simulink model "Doppelpendel_LQG"  (R2020b)
settings: Solver=ode45  StartTime=0.0  StopTime=10  EnableMultiTasking=on
values from neighbouring files (symbols this model uses):
  Beobachter_Rueckfuehrung = 0    [LoadParameter.m]
  Quantisierung = 0    [LoadParameter.m]
undefined symbols (not defined in the file or in its folder): parDP, parFF, parKAL, parLQR
libraries: cstblocks x3
settings Model: Creator=tg  LastModifiedBy=Armin Wessel
settings DataIOCC: LimitDataPoints=on  SaveFormat=Array  SignalLoggingSaveFormat=ModelDataLogs  ReturnWorkspaceOutputs=off
settings OptimizationCC: ExpressionDepthLimit=2147483647  InitFltsAndDblsToZero=on  LifeSpan=inf
settings DebuggingCC: UnderspecifiedInitializationDetection=Classic  MergeDetectMultiDrivingBlocksExec=none  SolverPrmCheckMsg=warning  FcnCallInpInsideContextMsg=warning  AllowSymbolicDim=off  StateNameClashWarn=warning  SFUnexpectedBacktrackingDiag=warning  SFNoUnconditionalDefaultTransitionDiag=warning  SFExecutionAtInitializationDiag=none  ArithmeticOperatorsInVariantConditions=warning
settings HardwareCC: ProdBitPerPointer=32  ProdBitPerSizeT=32  ProdBitPerPtrDiffT=32  ProdLargestAtomicFloat=None  ProdIntDivRoundTo=Undefined  ProdEndianess=Unspecified  ProdWordSize=32  ProdHWDeviceType=32-bit Generic
settings ModelReferenceCC: PropagateSignalLabelsOutOfModel=off
settings SFSimCC: SimUseLocalCustomCode=off  SimParseCustomCode=off  CustomCodeUndefinedFunction=UseInterfaceOnly
settings RTWCC: RTWUseLocalCustomCode=off
settings CodeAppCC: StateflowObjectComments=on
settings GRTTargetCC: TargetLangStandard=C89/C90 (ANSI)  CombineOutputUpdateFcns=off  GRTInterface=on
settings ConfigComp: CovMetricSettings=dw  CovSaveCumulativeToWorkspaceVar=on  CovSaveSingleToWorkspaceVar=on  CovExternalEMLEnable=off

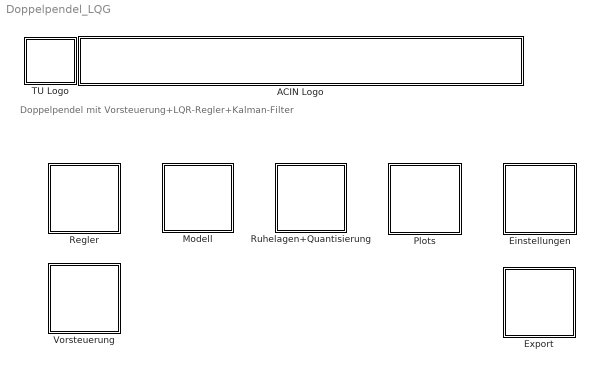
== system Doppelpendel_LQG ==
  note: Doppelpendel mit Vorsteuerung+LQR-Regler+Kalman-Filter
  ACIN Logo : Subsystem
      mask init:
      | s = get_param(gcb,'UserData');
      mask Display:
      | image(s.logo,[0 0 439 45]);
      | %axis image
  Einstellungen : Subsystem
  Export : Subsystem
  Modell : Subsystem
  Plots : Subsystem
  Regler : Subsystem
  Ruhelagen+Quantisierung : Subsystem
  TU Logo : Subsystem
      mask init:
      | s = get_param(gcb,'UserData');
      mask Display: image(s.logo,[0 0 45 45]);
  Vorsteuerung : Subsystem

== system Doppelpendel_LQG/ACIN Logo ==

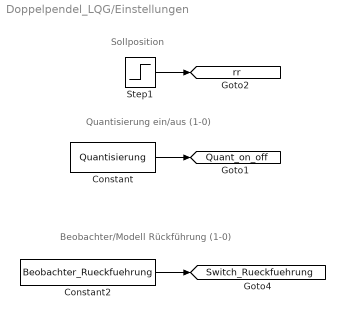
== system Doppelpendel_LQG/Einstellungen ==
  note: Sollposition
  note: Quantisierung ein/aus (1-0)
  note: Beobachter/Modell Rückführung (1-0)
  Constant : Constant  Value=Quantisierung
  Constant2 : Constant  Value=Beobachter_Rueckfuehrung
  Step1 : Step  After=0  SampleTime=parLQR.Ta
  tag scope: Quant_on_off=global, Switch_Rueckfuehrung=global, rr=global
  wires:
  Step1/1 -> [rr]
  Constant/1 -> [Quant_on_off]
  Constant2/1 -> [Switch_Rueckfuehrung]

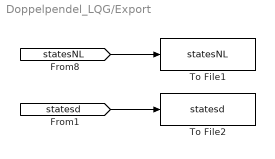
== system Doppelpendel_LQG/Export ==
  To File1 : ToFile  Filename=statesNL  MatrixName=data  SampleTime=parDP.Ta
  To File2 : ToFile  Filename=statesd  MatrixName=data  SampleTime=parDP.Ta
  wires:
  [statesNL] -> To File1/1
  [statesd] -> To File2/1

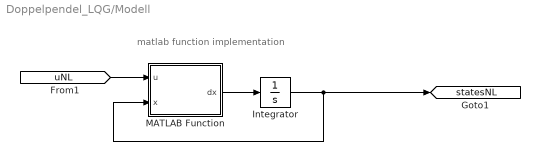
== system Doppelpendel_LQG/Modell ==
  note: matlab function implementation
  Integrator : Integrator  InitialCondition=parDP.IC
  MATLAB Function : MATLAB Function  TreatAsAtomicUnit=on
  tag scope: statesNL=global
  wires:
  [uNL] -> MATLAB Function/1(u)
  Integrator/1 -> [statesNL], MATLAB Function/2(x)
  MATLAB Function/1(dx) -> Integrator/1

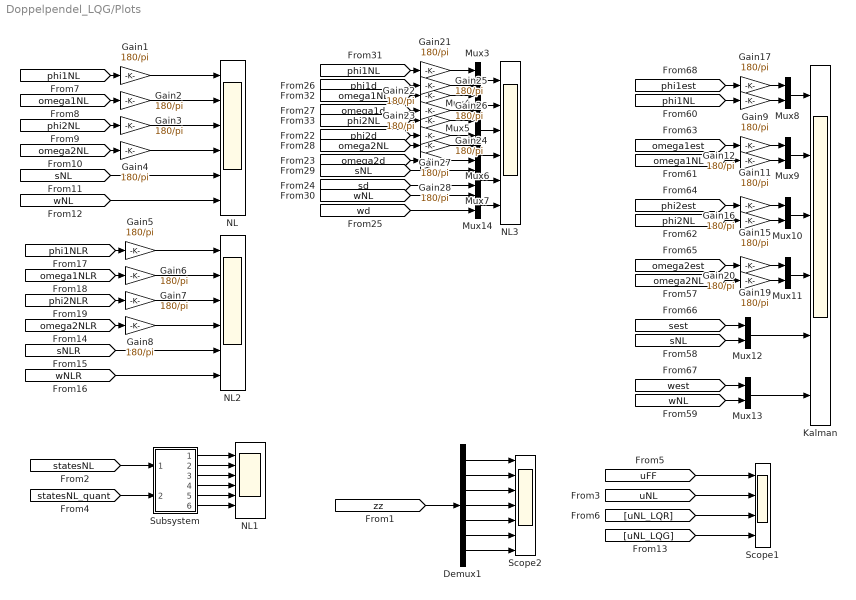
== system Doppelpendel_LQG/Plots ==
  Demux1 : Demux  Outputs=7
  Gain{1..9,11..12,15..17,19..28} (24 alike) : Gain  Gain=180/pi
  Kalman : Scope  NumInputPorts=6
  Mux{3..14} (12 alike) : Mux  Inputs=2
  NL{,1..3} (4 alike) : Scope  NumInputPorts=6
  Scope1 : Scope  NumInputPorts=4
  Scope2 : Scope  NumInputPorts=7
  Subsystem : Subsystem
  wires:
  [omega1NL] -> Gain2/1
  [omega2NL] -> Gain4/1
  [sNL] -> NL/5
  [wNL] -> NL/6
  Gain1/1 -> NL/1
  Gain2/1 -> NL/2
  Gain3/1 -> NL/3
  Gain4/1 -> NL/4
  [phi1NL] -> Gain1/1
  [phi2NL] -> Gain3/1
  [statesNL] -> Subsystem/1(In1)
  [statesNL_quant] -> Subsystem/2(In2)
  Subsystem/1(Out1) -> NL1/1
  Subsystem/2(Out2) -> NL1/2
  Subsystem/3(Out3) -> NL1/3
  Subsystem/4(Out4) -> NL1/4
  Subsystem/5(Out5) -> NL1/5
  Subsystem/6(Out6) -> NL1/6
  [omega1NL] -> Gain22/1
  [omega2NL] -> Gain24/1
  [phi1NL] -> Gain21/1
  [phi2NL] -> Gain23/1
  Mux3/1 -> NL3/1
  Mux4/1 -> NL3/2
  Mux5/1 -> NL3/3
  Mux6/1 -> NL3/4
  Mux7/1 -> NL3/5
  Mux14/1 -> NL3/6
  Gain21/1 -> Mux3/1
  Gain22/1 -> Mux4/1
  Gain23/1 -> Mux5/1
  Gain24/1 -> Mux6/1
  [sNL] -> Mux7/1
  [wNL] -> Mux14/1
  [phi1d] -> Gain25/1
  [omega1d] -> Gain26/1
  [phi2d] -> Gain27/1
  [omega2d] -> Gain28/1
  Gain25/1 -> Mux3/2
  Gain26/1 -> Mux4/2
  Gain27/1 -> Mux5/2
  Gain28/1 -> Mux6/2
  [sd] -> Mux7/2
  [wd] -> Mux14/2
  Demux1/1 -> Scope2/1
  Demux1/2 -> Scope2/2
  Demux1/3 -> Scope2/3
  Demux1/4 -> Scope2/4
  Demux1/5 -> Scope2/5
  Demux1/6 -> Scope2/6
  Demux1/7 -> Scope2/7
  [zz] -> Demux1/1
  Mux13/1 -> Kalman/6
  Mux12/1 -> Kalman/5
  Mux11/1 -> Kalman/4
  [omega1NL] -> Gain12/1
  [omega2NL] -> Gain20/1
  [phi1NL] -> Gain9/1
  [phi2NL] -> Gain16/1
  [sest] -> Mux12/1
  [west] -> Mux13/1
  [sNL] -> Mux12/2
  [wNL] -> Mux13/2
  Gain9/1 -> Mux8/2
  Gain17/1 -> Mux8/1
  [phi1est] -> Gain17/1
  Mux8/1 -> Kalman/1
  Gain12/1 -> Mux9/2
  Gain11/1 -> Mux9/1
  Mux9/1 -> Kalman/2
  [omega1est] -> Gain11/1
  Gain16/1 -> Mux10/2
  Gain15/1 -> Mux10/1
  [phi2est] -> Gain15/1
  Mux10/1 -> Kalman/3
  Gain20/1 -> Mux11/2
  Gain19/1 -> Mux11/1
  [omega2est] -> Gain19/1
  [uFF] -> Scope1/1
  [uNL] -> Scope1/2
  [uNL_LQR] -> Scope1/3
  [uNL_LQG] -> Scope1/4
  [omega1NLR] -> Gain6/1
  [omega2NLR] -> Gain8/1
  [sNLR] -> NL2/5
  [wNLR] -> NL2/6
  Gain5/1 -> NL2/1
  Gain6/1 -> NL2/2
  Gain7/1 -> NL2/3
  Gain8/1 -> NL2/4
  [phi1NLR] -> Gain5/1
  [phi2NLR] -> Gain7/1

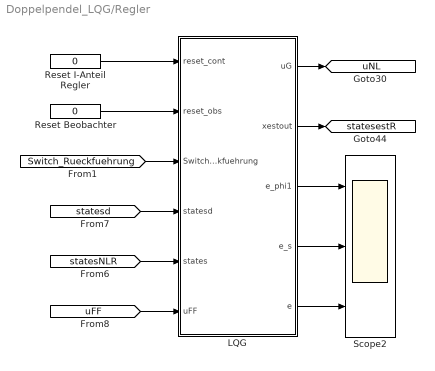
== system Doppelpendel_LQG/Regler ==
  LQG : MATLAB Function  TreatAsAtomicUnit=on
  Reset Beobachter : Constant  Value=0
  Reset I-Anteil Regler : Constant  Value=0
  Scope2 : Scope  NumInputPorts=3
  tag scope: statesestR=global, uNL=global
  wires:
  LQG/3(e_phi1) -> Scope2/1
  LQG/4(e_s) -> Scope2/2
  LQG/5(e) -> Scope2/3
  [statesNLR] -> LQG/5(states)
  LQG/2(xestout) -> [statesestR]
  [statesd] -> LQG/4(statesd)
  [uFF] -> LQG/6(uFF)
  LQG/1(uG) -> [uNL]
  Reset Beobachter/1 -> LQG/2(reset_obs)
  Reset I-Anteil Regler/1 -> LQG/1(reset_cont)
  [Switch_Rueckfuehrung] -> LQG/3(Switch_Rueckfuehrung)

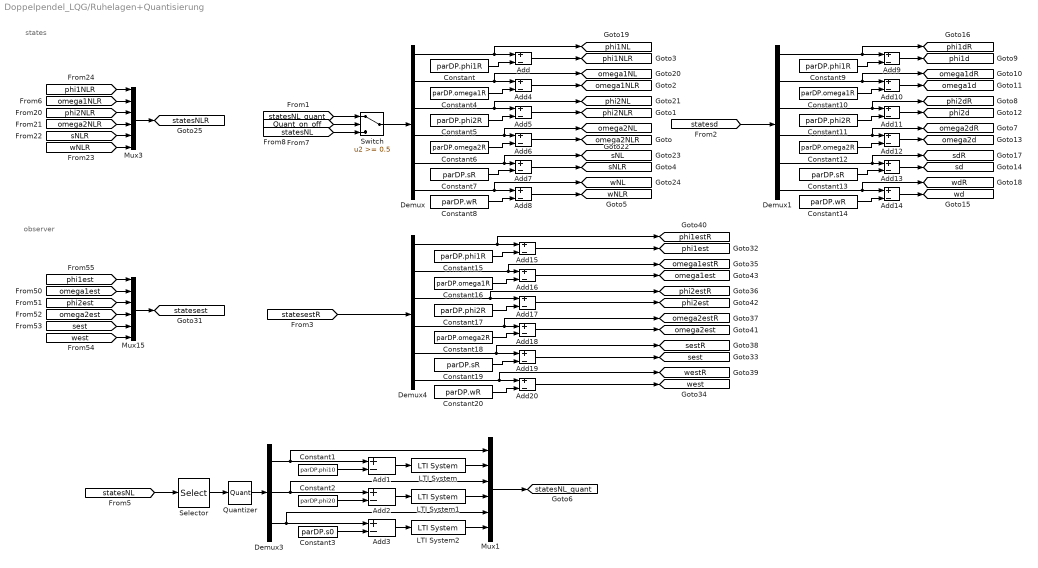
== system Doppelpendel_LQG/Ruhelagen+Quantisierung ==
  note: observer
  note: states
  Add{,1..20} (21 alike) : Sum  Inputs=+-
  Constant : Constant  Value=parDP.phi1R
  Constant1 : Constant  Value=parDP.phi10
  Constant10 : Constant  Value=parDP.omega1R
  Constant11 : Constant  Value=parDP.phi2R
  Constant12 : Constant  Value=parDP.omega2R
  Constant13 : Constant  Value=parDP.sR
  Constant14 : Constant  Value=parDP.wR
  Constant15 : Constant  Value=parDP.phi1R
  Constant16 : Constant  Value=parDP.omega1R
  Constant17 : Constant  Value=parDP.phi2R
  Constant18 : Constant  Value=parDP.omega2R
  Constant19 : Constant  Value=parDP.sR
  Constant2 : Constant  Value=parDP.phi20
  Constant20 : Constant  Value=parDP.wR
  Constant3 : Constant  Value=parDP.s0
  Constant4 : Constant  Value=parDP.omega1R
  Constant5 : Constant  Value=parDP.phi2R
  Constant6 : Constant  Value=parDP.omega2R
  Constant7 : Constant  Value=parDP.sR
  Constant8 : Constant  Value=parDP.wR
  Constant9 : Constant  Value=parDP.phi1R
  Demux : Demux  Outputs=6
  Demux1 : Demux  Outputs=6
  Demux3 : Demux  Outputs=3
  Demux4 : Demux  Outputs=6
  LTI System : cstblocks/LTI System  sys=Fd_diff  IC=[]
  LTI System1 : cstblocks/LTI System  sys=Fd_diff  IC=[]
  LTI System2 : cstblocks/LTI System  sys=Fd_diff  IC=[]
  Mux1 : Mux  Inputs=6
  Mux15 : Mux  Inputs=6
  Mux3 : Mux  Inputs=6
  Quantizer : Quantizer  QuantizationInterval=Phiquantisierung  SampleTime=parLQR.Ta
  Selector : Selector  InputPortWidth=6  IndexOptions=Index vector (dialog)  Indices=[1 3 5]  OutputSizes=1
  Switch : Switch  Threshold=0.5
  tag scope: omega1NL=global, omega1NLR=global, omega1d=global, omega1dR=global, omega1est=global, omega1estR=global, omega2NL=global, omega2NLR=global, omega2d=global, omega2dR=global, omega2est=global, omega2estR=global, phi1NL=global, phi1NLR=global, phi1d=global, phi1dR=global, phi1est=global, phi1estR=global, phi2NL=global, phi2NLR=global, phi2d=global, phi2dR=global, phi2est=global, phi2estR=global, sNL=global, sNLR=global, sd=global, sdR=global, sest=global, sestR=global, statesNLR=global, statesNL_quant=global, statesest=global, wNL=global, wNLR=global, wd=global, wdR=global, west=global, westR=global
  wires:
  [phi1NLR] -> Mux3/1
  [omega1NLR] -> Mux3/2
  [phi2NLR] -> Mux3/3
  [omega2NLR] -> Mux3/4
  [sNLR] -> Mux3/5
  [wNLR] -> Mux3/6
  Mux3/1 -> [statesNLR]
  [phi1est] -> Mux15/1
  [omega1est] -> Mux15/2
  [phi2est] -> Mux15/3
  [omega2est] -> Mux15/4
  [sest] -> Mux15/5
  [west] -> Mux15/6
  Mux15/1 -> [statesest]
  [statesNL] -> Selector/1
  Mux1/1 -> [statesNL_quant]
  LTI System/1 -> Mux1/2
  LTI System2/1 -> Mux1/6
  LTI System1/1 -> Mux1/4
  Add1/1 -> LTI System/1
  Add2/1 -> LTI System1/1
  Add3/1 -> LTI System2/1
  Constant1/1 -> Add1/2
  Constant2/1 -> Add2/2
  Constant3/1 -> Add3/2
  Demux3/3 -> Add3/1, Mux1/5
  Demux3/2 -> Add2/1, Mux1/3
  Demux3/1 -> Add1/1, Mux1/1
  [statesestR] -> Demux4/1
  Switch/1 -> Demux/1
  [Quant_on_off] -> Switch/2
  [statesNL_quant] -> Switch/1
  [statesNL] -> Switch/3
  [statesd] -> Demux1/1
  Quantizer/1 -> Demux3/1
  Selector/1 -> Quantizer/1
  Demux/1 -> [phi1NL], Add/1
  Constant4/1 -> Add4/2
  Demux/2 -> [omega1NL], Add4/1
  Add5/1 -> [phi2NLR]
  Add7/1 -> [sNLR]
  Constant7/1 -> Add7/2
  Constant5/1 -> Add5/2
  Add8/1 -> [wNLR]
  Constant6/1 -> Add6/2
  Demux/6 -> [wNL], Add8/1
  Demux/4 -> [omega2NL], Add6/1
  Add4/1 -> [omega1NLR]
  Constant8/1 -> Add8/2
  Add/1 -> [phi1NLR]
  Demux/3 -> [phi2NL], Add5/1
  Add6/1 -> [omega2NLR]
  Constant/1 -> Add/2
  Demux/5 -> [sNL], Add7/1
  Demux1/1 -> [phi1dR], Add9/1
  Constant10/1 -> Add10/2
  Demux1/2 -> [omega1dR], Add10/1
  Add11/1 -> [phi2d]
  Add13/1 -> [sd]
  Constant13/1 -> Add13/2
  Constant11/1 -> Add11/2
  Add14/1 -> [wd]
  Constant12/1 -> Add12/2
  Demux1/6 -> [wdR], Add14/1
  Demux1/4 -> [omega2dR], Add12/1
  Add10/1 -> [omega1d]
  Constant14/1 -> Add14/2
  Add9/1 -> [phi1d]
  Demux1/3 -> [phi2dR], Add11/1
  Add12/1 -> [omega2d]
  Constant9/1 -> Add9/2
  Demux1/5 -> [sdR], Add13/1
  Demux4/1 -> [phi1estR], Add15/1
  Constant16/1 -> Add16/2
  Demux4/2 -> [omega1estR], Add16/1
  Add17/1 -> [phi2est]
  Add19/1 -> [sest]
  Constant19/1 -> Add19/2
  Constant17/1 -> Add17/2
  Add20/1 -> [west]
  Constant18/1 -> Add18/2
  Demux4/6 -> Add20/1, [westR]
  Demux4/4 -> Add18/1, [omega2estR]
  Add16/1 -> [omega1est]
  Constant20/1 -> Add20/2
  Add15/1 -> [phi1est]
  Demux4/3 -> Add17/1, [phi2estR]
  Add18/1 -> [omega2est]
  Constant15/1 -> Add15/2
  Demux4/5 -> Add19/1, [sestR]

== system Doppelpendel_LQG/TU Logo ==

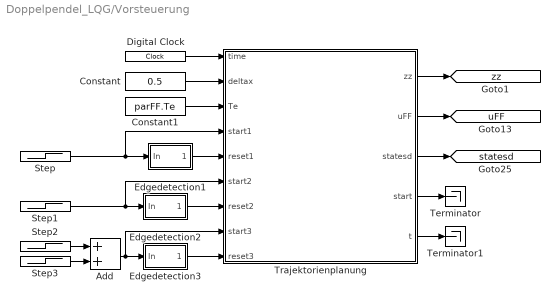
== system Doppelpendel_LQG/Vorsteuerung ==
  Add : Sum
  Constant : Constant  Value=0.5
  Constant1 : Constant  Value=parFF.Te
  Digital Clock : DigitalClock  SampleTime=parLQR.Ta
  Edgedetection1 : Subsystem
  Edgedetection2 : Subsystem
  Edgedetection3 : Subsystem
  Step : Step  Time=2  SampleTime=0
  Step1 : Step  Time=6  SampleTime=0
  Step2 : Step  Time=14  After=-1  SampleTime=0
  Step3 : Step  Time=10  SampleTime=0
  Terminator : Terminator
  Terminator1 : Terminator
  Trajektorienplanung : MATLAB Function  TreatAsAtomicUnit=on
  tag scope: statesd=global, uFF=global, zz=global
  wires:
  Trajektorienplanung/1(zz) -> [zz]
  Trajektorienplanung/5(t) -> Terminator1/1
  Trajektorienplanung/4(start) -> Terminator/1
  Step3/1 -> Add/2
  Step2/1 -> Add/1
  Edgedetection3/1(Out1) -> Trajektorienplanung/9(reset3)
  Step1/1 -> Edgedetection2/1(In), Trajektorienplanung/6(start2)
  Edgedetection2/1(Out1) -> Trajektorienplanung/7(reset2)
  Edgedetection1/1(Out1) -> Trajektorienplanung/5(reset1)
  Digital Clock/1 -> Trajektorienplanung/1(time)
  Trajektorienplanung/3(statesd) -> [statesd]
  Step/1 -> Edgedetection1/1(In), Trajektorienplanung/4(start1)
  Trajektorienplanung/2(uFF) -> [uFF]
  Constant/1 -> Trajektorienplanung/2(deltax)
  Constant1/1 -> Trajektorienplanung/3(Te)
  Add/1 -> Edgedetection3/1(In), Trajektorienplanung/8(start3)

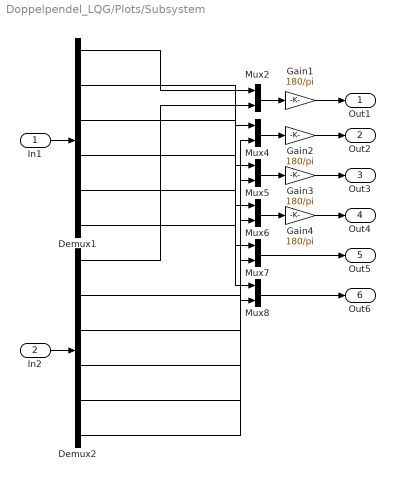
== system Doppelpendel_LQG/Plots/Subsystem ==
  In1 : Inport
  In2 : Inport  Port=2
  Demux1 : Demux  Outputs=6
  Demux2 : Demux  Outputs=6
  Gain{1..4} (4 alike) : Gain  Gain=180/pi
  Mux{2,4..8} (6 alike) : Mux  Inputs=2
  Out1 : Outport  VectorParamsAs1DForOutWhenUnconnected=off
  Out2 : Outport  Port=2  VectorParamsAs1DForOutWhenUnconnected=off
  Out3 : Outport  Port=3  VectorParamsAs1DForOutWhenUnconnected=off
  Out4 : Outport  Port=4  VectorParamsAs1DForOutWhenUnconnected=off
  Out5 : Outport  Port=5  VectorParamsAs1DForOutWhenUnconnected=off
  Out6 : Outport  Port=6  VectorParamsAs1DForOutWhenUnconnected=off
  wires:
  Demux1/1 -> Mux2/1
  Demux2/1 -> Mux2/2
  Demux2/2 -> Mux4/2
  Demux2/3 -> Mux5/2
  Demux2/4 -> Mux6/2
  Demux2/5 -> Mux7/2
  Demux2/6 -> Mux8/2
  Demux1/6 -> Mux8/1
  Demux1/5 -> Mux7/1
  Demux1/2 -> Mux4/1
  Demux1/3 -> Mux5/1
  Demux1/4 -> Mux6/1
  Mux2/1 -> Gain1/1
  Mux4/1 -> Gain2/1
  In1/1 -> Demux1/1
  Mux5/1 -> Gain3/1
  Mux6/1 -> Gain4/1
  Mux7/1 -> Out5/1
  Mux8/1 -> Out6/1
  In2/1 -> Demux2/1
  Gain1/1 -> Out1/1
  Gain2/1 -> Out2/1
  Gain3/1 -> Out3/1
  Gain4/1 -> Out4/1

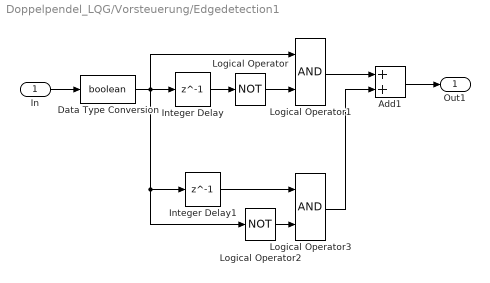
== system Doppelpendel_LQG/Vorsteuerung/Edgedetection1 ==
  In : Inport
  Add1 : Sum
  Data Type Conversion : DataTypeConversion  OutDataTypeStr=boolean  SaturateOnIntegerOverflow=on  RndMeth=Zero
  Integer Delay : Delay  DelayLength=1  SampleTime=parLQR.Ta
  Integer Delay1 : Delay  DelayLength=1  SampleTime=parLQR.Ta
  Logical Operator : Logic  Operator=NOT  Inputs=1
  Logical Operator1 : Logic
  Logical Operator2 : Logic  Operator=NOT  Inputs=1
  Logical Operator3 : Logic
  Out1 : Outport  VectorParamsAs1DForOutWhenUnconnected=off
  wires:
  In/1 -> Data Type Conversion/1
  Integer Delay/1 -> Logical Operator/1
  Data Type Conversion/1 -> Logical Operator1/1, Integer Delay/1, Integer Delay1/1, Logical Operator2/1
  Logical Operator/1 -> Logical Operator1/2
  Logical Operator2/1 -> Logical Operator3/2
  Integer Delay1/1 -> Logical Operator3/1
  Logical Operator1/1 -> Add1/1
  Logical Operator3/1 -> Add1/2
  Add1/1 -> Out1/1

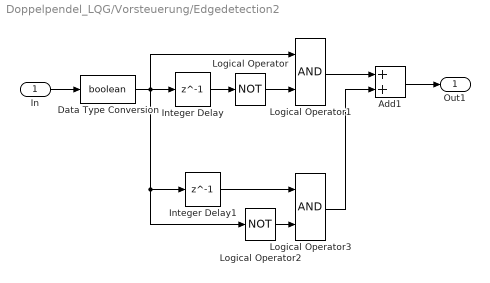
== system Doppelpendel_LQG/Vorsteuerung/Edgedetection2 ==
  In : Inport
  Add1 : Sum
  Data Type Conversion : DataTypeConversion  OutDataTypeStr=boolean  SaturateOnIntegerOverflow=on  RndMeth=Zero
  Integer Delay : Delay  DelayLength=1  SampleTime=parLQR.Ta
  Integer Delay1 : Delay  DelayLength=1  SampleTime=parLQR.Ta
  Logical Operator : Logic  Operator=NOT  Inputs=1
  Logical Operator1 : Logic
  Logical Operator2 : Logic  Operator=NOT  Inputs=1
  Logical Operator3 : Logic
  Out1 : Outport  VectorParamsAs1DForOutWhenUnconnected=off
  wires:
  Add1/1 -> Out1/1
  Logical Operator3/1 -> Add1/2
  Logical Operator1/1 -> Add1/1
  Integer Delay1/1 -> Logical Operator3/1
  Logical Operator2/1 -> Logical Operator3/2
  Logical Operator/1 -> Logical Operator1/2
  Data Type Conversion/1 -> Logical Operator2/1, Integer Delay1/1, Integer Delay/1, Logical Operator1/1
  Integer Delay/1 -> Logical Operator/1
  In/1 -> Data Type Conversion/1

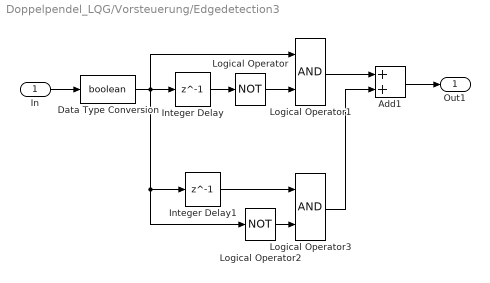
== system Doppelpendel_LQG/Vorsteuerung/Edgedetection3 ==
  In : Inport
  Add1 : Sum
  Data Type Conversion : DataTypeConversion  OutDataTypeStr=boolean  SaturateOnIntegerOverflow=on  RndMeth=Zero
  Integer Delay : Delay  DelayLength=1  SampleTime=parLQR.Ta
  Integer Delay1 : Delay  DelayLength=1  SampleTime=parLQR.Ta
  Logical Operator : Logic  Operator=NOT  Inputs=1
  Logical Operator1 : Logic
  Logical Operator2 : Logic  Operator=NOT  Inputs=1
  Logical Operator3 : Logic
  Out1 : Outport  VectorParamsAs1DForOutWhenUnconnected=off
  wires:
  In/1 -> Data Type Conversion/1
  Integer Delay/1 -> Logical Operator/1
  Data Type Conversion/1 -> Logical Operator1/1, Integer Delay/1, Integer Delay1/1, Logical Operator2/1
  Logical Operator/1 -> Logical Operator1/2
  Logical Operator2/1 -> Logical Operator3/2
  Integer Delay1/1 -> Logical Operator3/1
  Logical Operator1/1 -> Add1/1
  Logical Operator3/1 -> Add1/2
  Add1/1 -> Out1/1

== matlab function Doppelpendel_LQG/Modell/MATLAB Function ==
  data: u input; dx output; x input; parDP parameter
function dx = fcnDoppelpendel(u,x,parDP)
    %#codegen
    dx = Doppelpendel_NL_mfun(u,x,parDP);
end

== matlab function Doppelpendel_LQG/Regler/LQG ==
  settings: updateMethod=DISCRETE  sampleTime=parLQR.Ta
  data: reset_cont input; reset_obs input; Switch_Rueckfuehrung input; statesd input; states input; uFF input; uG output; parLQR parameter; xestout output; e_phi1 output; e_s output; parKAL parameter; e output
function [uG,xestout,e_phi1,e_s,e]  = LQG(reset_cont,reset_obs,Switch_Rueckfuehrung,statesd,states,uFF,parLQR,parKAL)

%Anfangsbedinungen
persistent xI
if isempty(xI) xI = double(0); end

persistent phi1est
if isempty(phi1est)phi1est = 0; end
persistent omega1est
if isempty(omega1est)omega1est = 0; end
persistent phi2est
if isempty(phi2est)phi2est = 0; end
persistent omega2est
if isempty(omega2est)omega2est = 0; end
persistent sest
if isempty(sest)sest = 0; end
persistent west
if isempty(west)west = 0; end

%Ausgang
xestout=[phi1est,omega1est,phi2est,omega2est,sest,west]';

%Beobachterrückführung ein/aus
if (Switch_Rueckfuehrung)
    xest=xestout;
else
    xest=states;
end
%%%%%%%%%%%%%%%%%%%%%%%%%%%%%%%%%%%%%%%%%%%%%%%%%%%%%%%%%%%%%%%%%%%%%%%%%%%
%LQR-Regler
%%%%%%%%%%%%%%%%%%%%%%%%%%%%%%%%%%%%%%%%%%%%%%%%%%%%%%%%%%%%%%%%%%%%%%%%%%%

% Folgendes hier bitte ausführen:
% 1.) PI-Zustandsregler einfügen
    % Integralschritt
    xI = xI + (statesd(5) - xest(5));
% 2.) if (reset_cont==1) xI=0 end
    if (reset_cont==1) 
    xI=0;
    end

%Gesamtrückführung
uFB = parLQR.kx*(xest - statesd) + parLQR.kI * xI; % Feedback Teil Regelung
uG = uFB + uFF; % Feedback und Feedforward
%%%%%%%%%%%%%%%%%%%%%%%%%%%%%%%%%%%%%%%%%%%%%%%%%%%%%%%%%%%%%%%%%%%%%%%%%%%
%Kalman-Filter
%%%%%%%%%%%%%%%%%%%%%%%%%%%%%%%%%%%%%%%%%%%%%%%%%%%%%%%%%%%%%%%%%%%%%%%%%%%

% Folgendes hier bitte ausführen:
% 1.) Kalman-Filter einfügen
    xest = parKAL.Asysd*xest + parKAL.bsysd*uG + parKAL.KK*([states(5); states(1)] - [ xest(5); xest(1)]);
    % states(5) = s
    % states(1) = phi1
    
% 2.) if (reset_obs==1) xestout=[0,0,0,0,0,0]' end
    if (reset_obs==1) 
        xestout = [0,0,0,0,0,0]';
    end
    
% 3.) xest befüllen
    phi1est = xest(1);
    omega1est = xest(2);
    phi2est = xest(3);
    omega2est = xest(4);
    sest = xest(5);
    west = xest(6);
    
% 4.) Fehlersystem befüllen
    e_phi1 = phi1est - states(1);
    e_s = sest - states(5);
    e =[e_phi1 ;0; 0; 0; e_s ;0];

== matlab function Doppelpendel_LQG/Vorsteuerung/Trajektorienplanung ==
  settings: updateMethod=DISCRETE  sampleTime=parLQR.Ta
  data: time input; deltax input; Te input; zz output; parFF parameter; uFF output; statesd output; start1 input; reset1 input; start2 input; start output; reset2 input; t output; start3 input; reset3 input
% Trajektorienplanung zum Versetzten des Doppelpendels
function [zz,uFF,statesd,start,t] = Trajektorienplanung(time,deltax,Te,parFF,start1,reset1,start2,reset2,start3,reset3)

persistent tstart
if isempty(tstart) tstart = double(0); end
persistent x0
if isempty(x0) x0 = double(0); end
persistent xT
if isempty(xT) xT = double(deltax); end


if reset1>0.5 || reset2>0.5 || reset3>0.5
    
    tstart = time;

end
%Zeit ab tstart
t = time - tstart;


if  start1>0.5 
    
    start = 1;
    
    if start2<0.5
        
        x0=0;
        xT=deltax; 
        
    else
        
        if start3<0.5
        
            x0=deltax;
            xT=-deltax; 
        
        else
    
            %Anfangs- und Endwert
            x0=-deltax;
            xT=deltax;
            
        end

    end
    
else
    
    start = 0;
    
end

% Folgendes hier bitte ausführen:
% 1.) Umrechnung auf Anfangs- und Endwert des Flachen Ausgangs
% 2.) Funktion Trajektorie() ergänzen
% 3.) Vorsteuerungsberechnung uFF ergänzen
% 4.) Sollzustandsverlauf statesd ergänzen

%Umrechnung auf Anfangs- und Endwert des Flachen Ausgangs
VV = inv(parFF.VVinv);
z0 = VV*x0;
zT = VV*xT;

z0 = z0(1);
zT = zT(1);

zz = Trajektorie(start,t,Te,z0,zT,parFF);
%zz=[z,zdot,z2dot,z3dot,z4dot,z5dot,z6dot];

%Vorsteuerung
uFF = parFF.aa' * zz';
%Sollzustandsverlauf
statesd =  parFF.VVinv * zz(1:6)';
end

%%%%%%%%%%%%%%%%%%%%%%%%%%%%%%%%%%%%%%%%%%%%%%%%%%%%%%%%%%%%%%%%%%%%%%%%%%    
function [zz] = Trajektorie(start,t,Te,z0,zT,parFF)
    
    if start<0.5

        z     = z0; 
        zdot  = 0; 
        z2dot = 0; 
        z3dot = 0; 
        z4dot = 0; 
        z5dot = 0; 
        z6dot = 0; 

    elseif start>0.5 && t<Te

        % Folgendes hier bitte ausführen:
        % 1.) Berechnung der Solltrajektorie
        beta_7 = parFF.beta7;
        beta_8 = parFF.beta8;
        beta_9 = parFF.beta9;
        beta_10 = parFF.beta10;
        beta_11 = parFF.beta11;
        beta_12 = parFF.beta12;
        beta_13 = parFF.beta13;
        Te = parFF.Te;

        zT_z0 = zT - z0;

        z = z0 + zT_z0 * (beta_7 * t ^ 7 / Te ^ 7 + beta_8 * t ^ 8 / Te ^ 8 + beta_9 * t ^ 9 / Te ^ 9 + beta_10 * t ^ 10 / Te ^ 10 + beta_11 * t ^ 11 / Te ^ 11 + beta_12 * t ^ 12 / Te ^ 12 + beta_13 * t ^ 13 / Te ^ 13);
        zdot = zT_z0 * (7 * beta_7 * t ^ 6 / Te ^ 7 + 8 * beta_8 * t ^ 7 / Te ^ 8 + 9 * beta_9 * t ^ 8 / Te ^ 9 + 10 * beta_10 * t ^ 9 / Te ^ 10 + 11 * beta_11 * t ^ 10 / Te ^ 11 + 12 * beta_12 * t ^ 11 / Te ^ 12 + 13 * beta_13 * t ^ 12 / Te ^ 13);
        z2dot = zT_z0 * (42 * beta_7 * t ^ 5 / Te ^ 7 + 56 * beta_8 * t ^ 6 / Te ^ 8 + 72 * beta_9 * t ^ 7 / Te ^ 9 + 90 * beta_10 * t ^ 8 / Te ^ 10 + 110 * beta_11 * t ^ 9 / Te ^ 11 + 132 * beta_12 * t ^ 10 / Te ^ 12 + 156 * beta_13 * t ^ 11 / Te ^ 13);
        z3dot = zT_z0 * (210 * beta_7 * t ^ 4 / Te ^ 7 + 336 * beta_8 * t ^ 5 / Te ^ 8 + 504 * beta_9 * t ^ 6 / Te ^ 9 + 720 * beta_10 * t ^ 7 / Te ^ 10 + 990 * beta_11 * t ^ 8 / Te ^ 11 + 1320 * beta_12 * t ^ 9 / Te ^ 12 + 1716 * beta_13 * t ^ 10 / Te ^ 13);
        z4dot = zT_z0 * (840 * beta_7 * t ^ 3 / Te ^ 7 + 1680 * beta_8 * t ^ 4 / Te ^ 8 + 3024 * beta_9 * t ^ 5 / Te ^ 9 + 5040 * beta_10 * t ^ 6 / Te ^ 10 + 7920 * beta_11 * t ^ 7 / Te ^ 11 + 11880 * beta_12 * t ^ 8 / Te ^ 12 + 17160 * beta_13 * t ^ 9 / Te ^ 13);
        z5dot = zT_z0 * (2520 * beta_7 * t ^ 2 / Te ^ 7 + 6720 * beta_8 * t ^ 3 / Te ^ 8 + 15120 * beta_9 * t ^ 4 / Te ^ 9 + 30240 * beta_10 * t ^ 5 / Te ^ 10 + 55440 * beta_11 * t ^ 6 / Te ^ 11 + 95040 * beta_12 * t ^ 7 / Te ^ 12 + 154440 * beta_13 * t ^ 8 / Te ^ 13);
        z6dot = zT_z0 * (5040 * beta_7 * t / Te ^ 7 + 20160 * beta_8 * t ^ 2 / Te ^ 8 + 60480 * beta_9 * t ^ 3 / Te ^ 9 + 151200 * beta_10 * t ^ 4 / Te ^ 10 + 332640 * beta_11 * t ^ 5 / Te ^ 11 + 665280 * beta_12 * t ^ 6 / Te ^ 12 + 1235520 * beta_13 * t ^ 7 / Te ^ 13);

        
    else

        z     = zT; 
        zdot  = 0; 
        z2dot = 0; 
        z3dot = 0; 
        z4dot = 0; 
        z5dot = 0; 
        z6dot = 0; 

    end

    zz=[z,zdot,z2dot,z3dot,z4dot,z5dot,z6dot];

end
